simulink model "Ldg_1a"  (R2021a)
settings: Solver=ode4  StartTime=0.0  StopTime=60.0  FixedStep=0.05  RelTol=1e-3
values from neighbouring files (symbols this model uses):
  A = 1.6    [LDG_1A_function.m]    (also in ODE2ndorder.m)
  B = 0.06    [LDG_1A_function.m]    (also in ODE2ndorder.m)
  gamma_0 = -140    [LDG_1A_function.m]
  Max_val = [Umax; Wmax; Xmax; Zmax; n_normax; n_tangmax]    [LDG_1A_function.m]
  Min_val = [Umin; Wmin; Xmin; Zmin; n_normin; n_tangmin]    [LDG_1A_function.m]
libraries: simulink x4
settings Model: Creator=stephanciobanu  LastModifiedBy=stephanciobanu

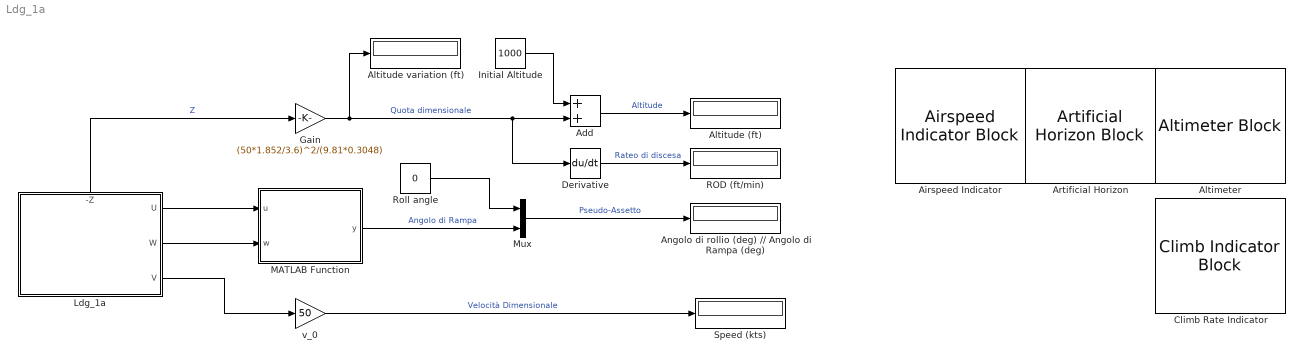
== system Ldg_1a ==
  Add : Sum
  Airspeed Indicator : AirspeedIndicatorBlock  LabelPosition=Hide  ScaleMin=0  ScaleMax=200
  Altimeter : AltimeterBlock  LabelPosition=Hide
  Altitude (ft) : Display
  Altitude variation (ft) : Display
  Angolo di rollio (deg) // Angolo di Rampa (deg) : Display
  Artificial Horizon : ArtificialHorizonBlock  LabelPosition=Hide
  Climb Rate Indicator : ClimbIndicatorBlock  LabelPosition=Hide  ScaleMax=1000
  Derivative : Derivative
  Gain : Gain  Gain=(50*1.852/3.6)^2/(9.81*0.3048)
  Initial Altitude : Constant  Value=1000
  Ldg_1a : Subsystem
      settings: PortSchema="{\"entries\":[{\"content\":{\"sides\":[{\"content\":{\"connectorIds\":[]},\"type\":\"ConnectorPlacement.EquallySpacedRectSide\",\"uuid\":\"4eeddddf-5648-4c88-8f7b-ba758a5b9acf\"},{\"content\":{\"connectorIds\":[\"Out1\",\"Out2\",\"Out3\"],\"side\":\"RIGHT\"},\"type\":\"ConnectorPlacement.EquallySpacedRectSide\",\"uuid\":\"a418b520-34c7-4937-9a68-89fd52b02874\"},{\"content\":{\"connectorIds\":[\"Out4\"],\"side\":\"TOP\"},\"type\":\"ConnectorPlacement.EquallySpacedRectSide\",\"uuid\":\"c96ecd47-a2ed-4de4-86a7-44412e6c5235\"}]},\"type\":\"ConnectorPlacement.EquallySpacedConnector\",\"uuid\":\"d5315b60-00cd-4f0a-be72-f1d8f91c931e\"}],\"packageUris\":[\"http://schema.mathworks.com/mf0/Connector/R2020b\"],\"version\":\"1.0\"}"
  MATLAB Function : MATLAB Function  TreatAsAtomicUnit=on
  Mux : Mux  Inputs=2
  ROD (ft/min) : Display
  Roll angle : Constant  Value=0
  Speed (kts) : Display
  v_0 : Gain  Gain=50
  wires:
  Mux/1 -> Angolo di rollio (deg) // Angolo di Rampa (deg)/1  "Pseudo-Assetto"
  Roll angle/1 -> Mux/1
  Ldg_1a/2(W) -> MATLAB Function/2(w)
  Ldg_1a/1(U) -> MATLAB Function/1(u)
  Ldg_1a/3(V) -> v_0/1
  Ldg_1a/4(-Z) -> Gain/1  "Z"
  Gain/1 -> Altitude variation (ft)/1, Add/2, Derivative/1  "Quota dimensionale"
  v_0/1 -> Speed (kts)/1  "Velocità Dimensionale"
  Initial Altitude/1 -> Add/1
  Add/1 -> Altitude (ft)/1  "Altitude"
  MATLAB Function/1(y) -> Mux/2  "Angolo di Rampa"
  Derivative/1 -> ROD (ft/min)/1  "Rateo di discesa"

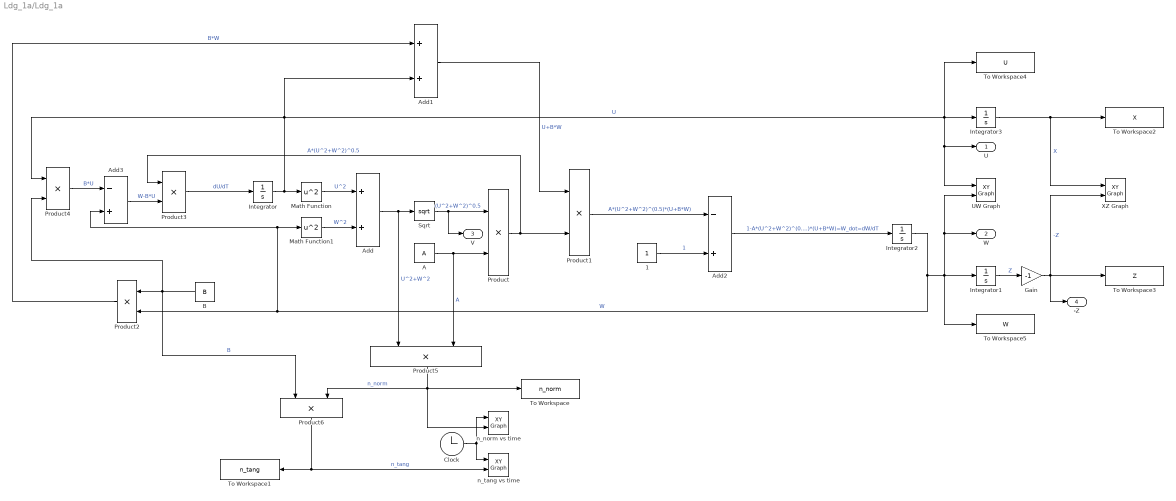
== system Ldg_1a/Ldg_1a ==
  1 : Constant
  A : Constant  Value=A
  Add : Sum
  Add1 : Sum
  Add2 : Sum  Inputs=-+
  Add3 : Sum  Inputs=-+
  B : Constant  Value=B
  Clock : Clock
  Gain : Gain  Gain=-1
  Integrator : Integrator  InitialCondition=cos(gamma_0*pi/180)
  Integrator1 : Integrator
  Integrator2 : Integrator  InitialCondition=-sin(gamma_0*pi/180)
  Integrator3 : Integrator
  Math Function : Math  Operator=square  SaturateOnIntegerOverflow=on
  Math Function1 : Math  Operator=square  SaturateOnIntegerOverflow=on
  Product{,1..6} (7 alike) : Product
  Sqrt : Sqrt  SaturateOnIntegerOverflow=on
  To Workspace : ToWorkspace  VariableName=n_norm  SaveFormat=Timeseries  SampleTime=-1
  To Workspace1 : ToWorkspace  VariableName=n_tang  SaveFormat=Timeseries  SampleTime=-1
  To Workspace2 : ToWorkspace  VariableName=X  SaveFormat=Timeseries  SampleTime=-1
  To Workspace3 : ToWorkspace  VariableName=Z  SaveFormat=Timeseries  SampleTime=-1
  To Workspace4 : ToWorkspace  VariableName=U  SaveFormat=Timeseries  SampleTime=-1
  To Workspace5 : ToWorkspace  VariableName=W  SaveFormat=Timeseries  SampleTime=-1
  UW Graph : simulink/Sinks/XY Graph  xmin=Min_val(1)  xmax=Max_val(1)  ymin=Min_val(2)  ymax=Max_val(2)  st=-1
  XZ Graph : simulink/Sinks/XY Graph  xmin=Min_val(3)  xmax=Max_val(3)  ymin=Min_val(4)  ymax=Max_val(4)  st=-1
  n_norm vs time : simulink/Sinks/XY Graph  xmin=0  xmax=60  ymin=Min_val(5)  ymax=Max_val(5)  st=-1
  n_tang vs time : simulink/Sinks/XY Graph  xmin=0  xmax=60  ymin=Min_val(6)  ymax=Max_val(6)  st=-1
  U : Outport
  W : Outport  Port=2
  V : Outport  Port=3
  -Z : Outport  Port=4
  wires:
  Integrator3/1 -> XZ Graph/1, To Workspace2/1  "X"
  Product4/1 -> Add3/1  "B*U"
  Product3/1 -> Integrator/1  "dU/dT"
  Clock/1 -> n_norm vs time/1, n_tang vs time/1
  Math Function/1 -> Add/1  "U^2"
  Add3/1 -> Product3/2  "W-B*U"
  Product1/1 -> Add2/1  "A*(U^2+W^2)^(0.5)*(U+B*W)"
  A/1 -> Product/2, Product5/2  "A"
  Product5/1 -> n_norm vs time/2, To Workspace/1, Product6/2  "n_norm"
  Integrator2/1 -> To Workspace5/1, UW Graph/2, W/1, Integrator1/1, Product2/2, Math Function1/1, Add3/2  "W"
  Integrator/1 -> Add1/2, Product4/1, U/1, UW Graph/1, Integrator3/1, To Workspace4/1, Math Function/1  "U"
  Add/1 -> Sqrt/1, Product5/1  "U^2+W^2"
  Integrator1/1 -> Gain/1  "Z"
  Product/1 -> Product3/1, Product1/2  "A*(U^2+W^2)^0.5"
  Gain/1 -> -Z/1, XZ Graph/2, To Workspace3/1  "-Z"
  Math Function1/1 -> Add/2  "W^2"
  Sqrt/1 -> V/1, Product/1  "(U^2+W^2)^0.5"
  Product2/1 -> Add1/1  "B*W"
  Add1/1 -> Product1/1  "U+B*W"
  Product6/1 -> To Workspace1/1, n_tang vs time/2  "n_tang"
  Add2/1 -> Integrator2/1  "1-A*(U^2+W^2)^(0.5)*(U+B*W)=W_dot=dW/dT"
  1/1 -> Add2/2  "1"
  B/1 -> Product4/2, Product2/1, Product6/1  "B"

== matlab function Ldg_1a/MATLAB Function ==
  data: u input; y output; w input
function y = angolo_rampa(u,w)

y = atan(-w/u)*180/pi;
